simulink subsystem "PvtSubSys_VSM_SCM"  (R2020b)
settings: Solver=VariableStepAuto  StartTime=0.0  StopTime=10.0  RelTol=1e-3
undefined symbols (not defined in the file): P_Global_VehicleWidthMin_m, P_VSM_LDW_State_Param_LaneTime, P_VSM_LDW_State_Param_Speed, P_VSM_LKA_State_Param_Offset, P_VSM_LSMC_SampleTime
libraries: simulink x45
(part 1 of 3)
settings Model: Creator=GW00199575  LastModifiedBy=GW00201118

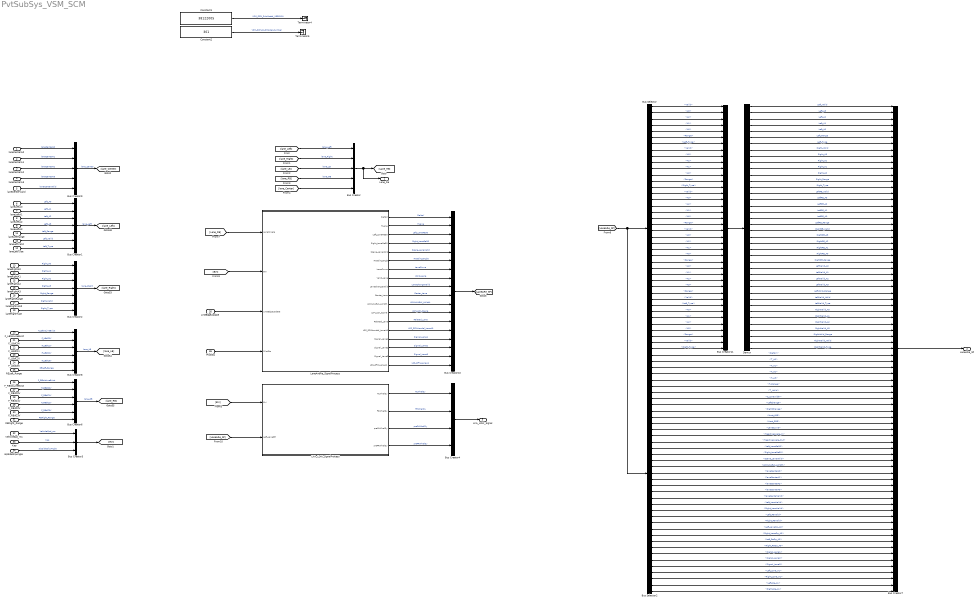
== system PvtSubSys_VSM_SCM ==
  laneCenterA0 : Inport
  laneCenterA1 : Inport  Port=2
  laneCenterA2 : Inport  Port=3
  laneCenterA3 : Inport  Port=4
  laneCenterValid : Inport  Port=5
  laneLeftA0 : Inport  Port=6
  laneLeftA1 : Inport  Port=7
  laneLeftA2 : Inport  Port=8
  laneLeftA3 : Inport  Port=9
  laneLeftValid : Inport  Port=10
  laneLeftRange : Inport  Port=11
  laneLeftType : Inport  Port=12
  laneRightA0 : Inport  Port=13
  laneRightA1 : Inport  Port=14
  laneRightA2 : Inport  Port=15
  laneRightA3 : Inport  Port=16
  laneRightValid : Inport  Port=17
  laneRightRange : Inport  Port=18
  laneRightType : Inport  Port=19
  F_LBbIsLineExist : Inport  Port=20
  F_LBdC0V : Inport  Port=21
  F_LBdC1V : Inport  Port=22
  F_LBdC2V : Inport  Port=23
  F_LBdC3V : Inport  Port=24
  RELeft_Range : Inport  Port=25
  F_RBbIsLineExist : Inport  Port=26
  F_RBdC0V : Inport  Port=27
  F_RBdC1V : Inport  Port=28
  F_RBdC2V : Inport  Port=29
  F_RBdC3V : Inport  Port=30
  RERight_Range : Inport  Port=31
  VehicleSpd_ms : Inport  Port=32
  Kap : Inport  Port=33
  alpSideSlipAngle : Inport  Port=34
  LIneEdgeUpdate : Inport  Port=35
  PilotSts : Inport  Port=36
  Bus Creator : BusCreator  Inputs=5
  Bus Creator1 : BusCreator  Inputs=7
  Bus Creator10 : BusCreator  Inputs=18
  Bus Creator11 : BusCreator  Inputs=40
  Bus Creator2 : BusCreator  Inputs=7
  Bus Creator3 : BusCreator  Inputs=3
  Bus Creator4 : BusCreator  Inputs=4
  Bus Creator6 : BusCreator  Inputs=6
  Bus Creator7 : BusCreator  Inputs=79
  Bus Creator8 : BusCreator  Inputs=6
  Bus Creator9 : BusCreator  Inputs=5
  Bus Selector : BusSelector  OutputSignals=HLane.Left_Lane.Valid,HLane.Left_Lane.A3,HLane.Left_Lane.A2,HLane.Left_Lane.A1,HLane.Left_Lane.A0,HLane.Left_Lane.Range,HLane.Left_Lane.Left_Type,HLane.Right_Lane.Valid,HLane.Right_Lane.A3,HLane.Right_Lane.A2,HLane.Right_Lane.A1,HLane.Right_Lane.A0,HLane.Right_Lane.Range,HLane.Right_Lane.Right_Type,HLane.Left_RE.Valid,HLane.Left_RE.A3,HLane.Left_RE.A2,HLane.Left_RE.A1,HLane.Left_RE.A0,HLane.Left_RE.Range,HLane.Right_RE.Valid,HLane.Right_RE.A3,HLane.Right_RE.A2,HLane.Right_RE.A1,HLane.Right_RE.A0,HLane.Right_RE.Range,Valid_Lane.Left_ValidLane.A0,Valid_Lane.Left_ValidLane.A1,Valid_Lane.Left_ValidLane.A2,Valid_Lane.Left_ValidLane.A3,Valid_Lane.Left_ValidLane.Range,Valid_Lane.Left_ValidLane.Valid,Valid_Lane.Left_ValidLane.Left_Type,Valid_Lane.Right_ValidLane.A0,Valid_Lane.Right_ValidLane.A1,Valid_Lane.Right_ValidLane.A2,Valid_Lane.Right_ValidLane.A3,Valid_Lane.Right_ValidLane.Range,Valid_Lane.Right_ValidLane.Valid,Valid_Lane.Right_ValidLane.Right_Type
  Bus Selector2 : BusSelector  OutputSignals=DeltaY,Center_Lane.T_A0,Center_Lane.T_A1,Center_Lane.T_A2,Center_Lane.T_A3,Center_Lane.T_Range,Center_Lane.T_Valid,Center_Lane.C_Lanewidth,LaneChangeValid.LeftChange,LaneChangeValid.RightChange,Valid_Lane.Host_LRE,Valid_Lane.Host_RRE,LaneCurve,Headingangle.HeadingAngle_In,Headingangle.HeadingAngle_Out,Left_LaneRe30,Right_LaneRe30,Scene_LaneValid,LDWLKAELK_LWidth,LSM_LCK_CLane.laneCenterA0,LSM_LCK_CLane.laneCenterA1,LSM_LCK_CLane.laneCenterA2,LSM_LCK_CLane.laneCenterA3,LSM_LCK_CLane.laneCenterValid,Related_Lane.Left_LaneValid,Related_Lane.Right_LaneValid,Related_Lane.Left_ReValid,Related_Lane.Right_ReValid,LSS_RFMHandel_LaneA0.Left_LaneOp_A0,LSS_RFMHandel_LaneA0.Right_LaneOp_A0,LSS_RFMHandel_LaneA0.Left_ReOp_A0,LSS_RFMHandel_LaneA0.Right_ReOp_A0,Signal_Lane1,Signal_Lane2,Signal_Lane3,LSS_RFM_LaneA1.Left_Lane_A1,LSS_RFM_LaneA1.Right_Lane_A1,LSS_RFM_LaneA1.Left_Re_A1,LSS_RFM_LaneA1.Right_Re_A1
  Constant1 : Constant  Value=38122005  OutDataTypeStr=uint32
  Constant2 : Constant  Value=301  OutDataTypeStr=uint16
  Demux : Demux  Outputs=40  BusSelectionMode=on
  LKA_LDW_SignalProcess : Subsystem
  LaneAndRe_SignalProcess : Subsystem
  Terminator4 : Terminator
  Terminator5 : Terminator
  Lane_Re : Outport
  LaneARe_SP : Outport  Port=2
  LKA_LDW_Signal : Outport  Port=3
  wires:
  Bus Selector2/39 -> Bus Creator7/79  "<Right_Re_A1>"
  Bus Selector2/38 -> Bus Creator7/78  "<Left_Re_A1>"
  Bus Selector2/37 -> Bus Creator7/77  "<Right_Lane_A1>"
  Bus Selector2/36 -> Bus Creator7/76  "<Left_Lane_A1>"
  Bus Selector2/35 -> Bus Creator7/75  "<Signal_Lane3>"
  Bus Selector2/34 -> Bus Creator7/74  "<Signal_Lane2>"
  Bus Selector2/33 -> Bus Creator7/73  "<Signal_Lane1>"
  Bus Selector2/32 -> Bus Creator7/72  "<Right_ReOp_A0>"
  Bus Selector2/31 -> Bus Creator7/71  "<Left_ReOp_A0>"
  Bus Selector2/30 -> Bus Creator7/70  "<Right_LaneOp_A0>"
  Bus Selector2/29 -> Bus Creator7/69  "<Left_LaneOp_A0>"
  Bus Selector2/28 -> Bus Creator7/68  "<Right_ReValid>"
  Bus Selector2/27 -> Bus Creator7/67  "<Left_ReValid>"
  Bus Selector2/26 -> Bus Creator7/66  "<Right_LaneValid>"
  Bus Selector2/25 -> Bus Creator7/65  "<Left_LaneValid>"
  Bus Selector2/24 -> Bus Creator7/64  "<laneCenterValid>"
  LaneAndRe_SignalProcess/18(LSS_RFM_LaneA1) -> Bus Creator10/18  "LSS_RFM_LaneA1"
  LaneAndRe_SignalProcess/17(Signal_Lane3) -> Bus Creator10/17  "Signal_Lane3"
  LaneAndRe_SignalProcess/16(Signal_Lane2) -> Bus Creator10/16  "Signal_Lane2"
  LaneAndRe_SignalProcess/15(Signal_Lane1) -> Bus Creator10/15  "Signal_Lane1"
  LaneAndRe_SignalProcess/14(LSS_RFMHandel_LaneA0) -> Bus Creator10/14  "LSS_RFMHandel_LaneA0"
  LaneAndRe_SignalProcess/13(Related_Lane) -> Bus Creator10/13  "Related_Lane"
  LaneAndRe_SignalProcess/12(LSM_LCK_CLane) -> Bus Creator10/12  "LSM_LCK_CLane"
  LaneAndRe_SignalProcess/11(LDWLKAELK_LWidth) -> Bus Creator10/11  "LDWLKAELK_LWidth"
  PilotSts/1 -> LaneAndRe_SignalProcess/4(PilotSts)
  [LaneARe_SP] -> LKA_LDW_SignalProcess/2(Left_LaneRE)
  [lane_Center] -> Bus Creator/5
  LKA_LDW_SignalProcess/4(preFRWhelDy) -> Bus Creator4/4  "preFRWhelDy"
  LKA_LDW_SignalProcess/3(preFLWhelDy) -> Bus Creator4/3  "preFLWhelDy"
  LKA_LDW_SignalProcess/2(FRWhelDy) -> Bus Creator4/2  "FRWhelDy"
  LKA_LDW_SignalProcess/1(FLWhelDy) -> Bus Creator4/1  "FLWhelDy"
  [EVI] -> LKA_LDW_SignalProcess/1(Evi)
  laneCenterValid/1 -> Bus Creator9/5  "laneCenterValid"
  Bus Creator9/1 -> [lane_Center]  "lane_Center"
  laneCenterA3/1 -> Bus Creator9/4  "laneCenterA3"
  laneCenterA0/1 -> Bus Creator9/1  "laneCenterA0"
  laneCenterA1/1 -> Bus Creator9/2  "laneCenterA1"
  laneCenterA2/1 -> Bus Creator9/3  "laneCenterA2"
  [EVI] -> LaneAndRe_SignalProcess/2(EVI)
  LIneEdgeUpdate/1 -> LaneAndRe_SignalProcess/3(LIneEdgeUpdate)
  [Lane_RE] -> LaneAndRe_SignalProcess/1(LaneSingle)
  LaneAndRe_SignalProcess/7(LaneCurve) -> Bus Creator10/7  "LaneCurve"
  LaneAndRe_SignalProcess/6(Headingangle) -> Bus Creator10/6  "Headingangle"
  LaneAndRe_SignalProcess/5(Scene_LaneValid) -> Bus Creator10/5  "Scene_LaneValid"
  Bus Creator10/1 -> [LaneARe_SP]
  LaneAndRe_SignalProcess/10(Center_Lane) -> Bus Creator10/10  "Center_Lane"
  LaneAndRe_SignalProcess/1(DeltaY) -> Bus Creator10/1  "DeltaY"
  LaneAndRe_SignalProcess/3(Left_LaneRe30) -> Bus Creator10/3  "Left_LaneRe30"
  LaneAndRe_SignalProcess/2(HLane) -> Bus Creator10/2  "HLane"
  LaneAndRe_SignalProcess/8(Valid_Lane) -> Bus Creator10/8  "Valid_Lane"
  LaneAndRe_SignalProcess/4(Right_LaneRe30) -> Bus Creator10/4  "Right_LaneRe30"
  LaneAndRe_SignalProcess/9(LaneChangeValid) -> Bus Creator10/9  "LaneChangeValid"
  laneRightType/1 -> Bus Creator2/7  "Right_Type"
  laneLeftType/1 -> Bus Creator1/7  "Left_Type"
  Bus Creator4/1 -> LKA_LDW_Signal/1
  Bus Creator3/1 -> [EVI]
  alpSideSlipAngle/1 -> Bus Creator3/3  "alpSideSlipAngle"
  Kap/1 -> Bus Creator3/2  "Kap"
  VehicleSpd_ms/1 -> Bus Creator3/1  "VehicleSpd_ms"
  Bus Creator/1 -> Lane_Re/1, [Lane_RE]
  [lane_RB] -> Bus Creator/4  "lane_RB"
  [lane_LB] -> Bus Creator/3  "lane_LB"
  [lane_Right] -> Bus Creator/2  "lane_Right"
  [lane_Left] -> Bus Creator/1  "lane_Left"
  Bus Creator6/1 -> [lane_RB]  "lane_RB"
  Bus Creator8/1 -> [lane_LB]  "lane_LB"
  Bus Creator2/1 -> [lane_Right]  "lane_Right"
  Bus Creator1/1 -> [lane_Left]  "lane_Left"
  RERight_Range/1 -> Bus Creator6/6  "RERight_Range"
  F_RBdC3V/1 -> Bus Creator6/5  "F_RBdC3V"
  F_RBdC2V/1 -> Bus Creator6/4  "F_RBdC2V"
  F_RBdC1V/1 -> Bus Creator6/3  "F_RBdC1V"
  F_RBdC0V/1 -> Bus Creator6/2  "F_RBdC0V"
  F_RBbIsLineExist/1 -> Bus Creator6/1  "F_RBbIsLineExist"
  RELeft_Range/1 -> Bus Creator8/6  "RELeft_Range"
  F_LBdC3V/1 -> Bus Creator8/5  "F_LBdC3V"
  F_LBdC2V/1 -> Bus Creator8/4  "F_LBdC2V"
  F_LBdC1V/1 -> Bus Creator8/3  "F_LBdC1V"
  F_LBdC0V/1 -> Bus Creator8/2  "F_LBdC0V"
  F_LBbIsLineExist/1 -> Bus Creator8/1  "F_LBbIsLineExist"
  laneRightValid/1 -> Bus Creator2/6  "Right_Valid"
  laneRightRange/1 -> Bus Creator2/5  "Right_Range"
  laneRightA0/1 -> Bus Creator2/1  "Right_A0"
  laneRightA3/1 -> Bus Creator2/4  "Right_A3"
  laneRightA1/1 -> Bus Creator2/2  "Right_A1"
  laneRightA2/1 -> Bus Creator2/3  "Right_A2"
  laneLeftValid/1 -> Bus Creator1/6  "Left_Valid"
  laneLeftRange/1 -> Bus Creator1/5  "Left_Range"
  laneLeftA2/1 -> Bus Creator1/3  "Left_A2"
  laneLeftA3/1 -> Bus Creator1/4  "Left_A3"
  laneLeftA1/1 -> Bus Creator1/2  "Left_A1"
  laneLeftA0/1 -> Bus Creator1/1  "Left_A0"
  [LaneARe_SP] -> Bus Selector/1, Bus Selector2/1
  Bus Creator7/1 -> LaneARe_SP/1
  Bus Selector/1 -> Bus Creator11/1  "<Valid>"
  Bus Selector/2 -> Bus Creator11/2  "<A3>"
  Bus Selector/3 -> Bus Creator11/3  "<A2>"
  Bus Selector/4 -> Bus Creator11/4  "<A1>"
  Bus Selector/5 -> Bus Creator11/5  "<A0>"
  Bus Selector/6 -> Bus Creator11/6  "<Range>"
  Bus Selector/7 -> Bus Creator11/7  "<Left_Type>"
  Bus Selector/8 -> Bus Creator11/8  "<Valid>"
  Bus Selector/9 -> Bus Creator11/9  "<A3>"
  Bus Selector/10 -> Bus Creator11/10  "<A2>"
  Bus Selector/11 -> Bus Creator11/11  "<A1>"
  Bus Selector/12 -> Bus Creator11/12  "<A0>"
  Bus Selector/13 -> Bus Creator11/13  "<Range>"
  Bus Selector/14 -> Bus Creator11/14  "<Right_Type>"
  Bus Selector/15 -> Bus Creator11/15  "<Valid>"
  Bus Selector/16 -> Bus Creator11/16  "<A3>"
  Bus Selector/17 -> Bus Creator11/17  "<A2>"
  Bus Selector/18 -> Bus Creator11/18  "<A1>"
  Bus Selector/19 -> Bus Creator11/19  "<A0>"
  Bus Selector/20 -> Bus Creator11/20  "<Range>"
  Bus Selector/21 -> Bus Creator11/21  "<Valid>"
  Bus Selector/22 -> Bus Creator11/22  "<A3>"
  Bus Selector/23 -> Bus Creator11/23  "<A2>"
  Bus Selector/24 -> Bus Creator11/24  "<A1>"
  Bus Selector/25 -> Bus Creator11/25  "<A0>"
  Bus Selector/26 -> Bus Creator11/26  "<Range>"
  Bus Selector/27 -> Bus Creator11/27  "<A0>"
  Bus Selector/28 -> Bus Creator11/28  "<A1>"
  Bus Selector/29 -> Bus Creator11/29  "<A2>"
  Bus Selector/30 -> Bus Creator11/30  "<A3>"
  Bus Selector/31 -> Bus Creator11/31  "<Range>"
  Bus Selector/32 -> Bus Creator11/32  "<Valid>"
  Bus Selector/33 -> Bus Creator11/33  "<Left_Type>"
  Bus Selector/34 -> Bus Creator11/34  "<A0>"
  Bus Selector/35 -> Bus Creator11/35  "<A1>"
  Bus Selector/36 -> Bus Creator11/36  "<A2>"
  Bus Selector/37 -> Bus Creator11/37  "<A3>"
  Bus Selector/38 -> Bus Creator11/38  "<Range>"
  Bus Selector/39 -> Bus Creator11/39  "<Valid>"
  Bus Selector/40 -> Bus Creator11/40  "<Right_Type>"
  Bus Creator11/1 -> Demux/1
  Demux/1 -> Bus Creator7/1  "Left_Valid"
  Demux/2 -> Bus Creator7/2  "Left_A3"
  Demux/3 -> Bus Creator7/3  "Left_A2"
  Demux/4 -> Bus Creator7/4  "Left_A1"
  Demux/5 -> Bus Creator7/5  "Left_A0"
  Demux/6 -> Bus Creator7/6  "Left_Range"
  Demux/7 -> Bus Creator7/7  "Left_Type"
  Demux/8 -> Bus Creator7/8  "Right_Valid"
  Demux/9 -> Bus Creator7/9  "Right_A3"
  Demux/10 -> Bus Creator7/10  "Right_A2"
  Demux/11 -> Bus Creator7/11  "Right_A1"
  Demux/12 -> Bus Creator7/12  "Right_A0"
  Demux/13 -> Bus Creator7/13  "Right_Range"
  Demux/14 -> Bus Creator7/14  "Right_Type"
  Demux/15 -> Bus Creator7/15  "LeftRE_Valid"
  Demux/16 -> Bus Creator7/16  "LeftRE_A3"
  Demux/17 -> Bus Creator7/17  "LeftRE_A2"
  Demux/18 -> Bus Creator7/18  "LeftRE_A1"
  Demux/19 -> Bus Creator7/19  "LeftRE_A0"
  Demux/20 -> Bus Creator7/20  "LeftRE_Range"
  Demux/21 -> Bus Creator7/21  "RightRE_Valid"
  Demux/22 -> Bus Creator7/22  "RightRE_A3"
  Demux/23 -> Bus Creator7/23  "RightRE_A2"
  Demux/24 -> Bus Creator7/24  "RightRE_A1"
  Demux/25 -> Bus Creator7/25  "RightRE_A0"
  Demux/26 -> Bus Creator7/26  "RightRE_Range"
  Demux/27 -> Bus Creator7/27  "LeftValid_A0"
  Demux/28 -> Bus Creator7/28  "LeftValid_A1"
  Demux/29 -> Bus Creator7/29  "LeftValid_A2"
  Demux/30 -> Bus Creator7/30  "LeftValid_A3"
  Demux/31 -> Bus Creator7/31  "LeftValid_Range"
  Demux/32 -> Bus Creator7/32  "LeftValid_Valid"
  Demux/33 -> Bus Creator7/33  "LeftValid_Type"
  Demux/34 -> Bus Creator7/34  "RightValid_A0"
  Demux/35 -> Bus Creator7/35  "RightValid_A1"
  Demux/36 -> Bus Creator7/36  "RightValid_A2"
  Demux/37 -> Bus Creator7/37  "RightValid_A3"
  Demux/38 -> Bus Creator7/38  "RightValid_Range"
  Demux/39 -> Bus Creator7/39  "RightValid_Valid"
  Demux/40 -> Bus Creator7/40  "RightValid_Type"
  Bus Selector2/1 -> Bus Creator7/41  "<DeltaY>"
  Bus Selector2/2 -> Bus Creator7/42  "<T_A0>"
  Bus Selector2/3 -> Bus Creator7/43  "<T_A1>"
  Bus Selector2/4 -> Bus Creator7/44  "<T_A2>"
  Bus Selector2/5 -> Bus Creator7/45  "<T_A3>"
  Bus Selector2/6 -> Bus Creator7/46  "<T_Range>"
  Bus Selector2/7 -> Bus Creator7/47  "<T_Valid>"
  Bus Selector2/8 -> Bus Creator7/48  "<C_Lanewidth>"
  Bus Selector2/9 -> Bus Creator7/49  "<LeftChange>"
  Bus Selector2/10 -> Bus Creator7/50  "<RightChange>"
  Bus Selector2/11 -> Bus Creator7/51  "<Host_LRE>"
  Bus Selector2/12 -> Bus Creator7/52  "<Host_RRE>"
  Bus Selector2/13 -> Bus Creator7/53  "<LaneCurve>"
  Bus Selector2/14 -> Bus Creator7/54  "<HeadingAngle_In>"
  Bus Selector2/15 -> Bus Creator7/55  "<HeadingAngle_Out>"
  Bus Selector2/16 -> Bus Creator7/56  "<Left_LaneRe30>"
  Bus Selector2/17 -> Bus Creator7/57  "<Right_LaneRe30>"
  Bus Selector2/18 -> Bus Creator7/58  "<Scene_LaneValid>"
  Bus Selector2/19 -> Bus Creator7/59  "<LDWLKAELK_LWidth>"
  Bus Selector2/20 -> Bus Creator7/60  "<laneCenterA0>"
  Bus Selector2/21 -> Bus Creator7/61  "<laneCenterA1>"
  Bus Selector2/22 -> Bus Creator7/62  "<laneCenterA2>"
  Bus Selector2/23 -> Bus Creator7/63  "<laneCenterA3>"
  Constant1/1 -> Terminator4/1  "VSM_SCM_SubModel_VERSION"
  Constant2/1 -> Terminator5/1  "VSM_SCM_SubModel_Number"

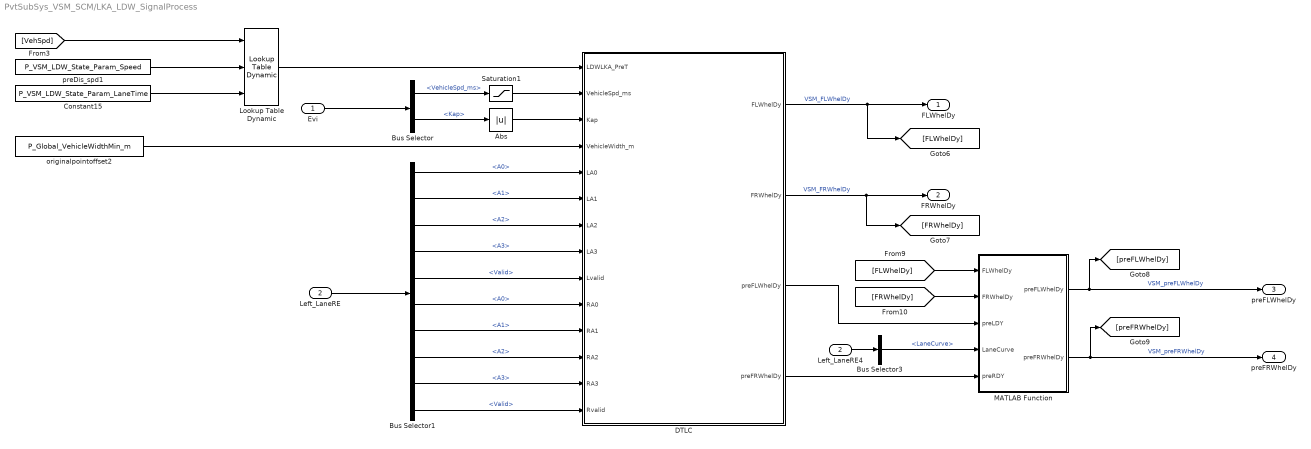
== system PvtSubSys_VSM_SCM/LKA_LDW_SignalProcess ==
  Evi : Inport
  Left_LaneRE : Inport  Port=2
  Abs : Abs
  Bus Selector : BusSelector  OutputSignals=VehicleSpd_ms,Kap
  Bus Selector1 : BusSelector  OutputSignals=Valid_Lane.Left_ValidLane.A0,Valid_Lane.Left_ValidLane.A1,Valid_Lane.Left_ValidLane.A2,Valid_Lane.Left_ValidLane.A3,Valid_Lane.Left_ValidLane.Valid,Valid_Lane.Right_ValidLane.A0,Valid_Lane.Right_ValidLane.A1,Valid_Lane.Right_ValidLane.A2,Valid_Lane.Right_ValidLane.A3,Valid_Lane.Right_ValidLane.Valid
  Bus Selector3 : BusSelector  OutputSignals=LaneCurve
  Constant15 : Constant  Value=P_VSM_LDW_State_Param_LaneTime
  DTLC : MATLAB Function  Description=%Lane inside is positive,outside is negitive  TreatAsAtomicUnit=on
  Left_LaneRE4 : InportShadow  Port=2
  Lookup Table Dynamic : simulink/Lookup Tables/Lookup Table Dynamic  LookUpMeth=Interpolation-Use End Values  OutDataType=fixdt('double')  OutScaling=[]  OutputDataTypeScalingMode=Specify via dialog  OutDataTypeStr=double  DoSatur=off
  MATLAB Function : MATLAB Function  TreatAsAtomicUnit=on
  Saturation1 : Saturate  UpperLimit=200  LowerLimit=0.001
  originalpointoffset2 : Constant  Value=P_Global_VehicleWidthMin_m
  preDis_spd1 : Constant  Value=P_VSM_LDW_State_Param_Speed
  FLWhelDy : Outport
  FRWhelDy : Outport  Port=2
  preFLWhelDy : Outport  Port=3
  preFRWhelDy : Outport  Port=4
  wires:
  Abs/1 -> DTLC/3(Kap)
  Bus Selector1/10 -> DTLC/14(Rvalid)  "<Valid>"
  Bus Selector1/9 -> DTLC/13(RA3)  "<A3>"
  Bus Selector1/8 -> DTLC/12(RA2)  "<A2>"
  Bus Selector1/7 -> DTLC/11(RA1)  "<A1>"
  Bus Selector1/6 -> DTLC/10(RA0)  "<A0>"
  originalpointoffset2/1 -> DTLC/4(VehicleWidth_m)
  Bus Selector1/5 -> DTLC/9(Lvalid)  "<Valid>"
  Bus Selector1/4 -> DTLC/8(LA3)  "<A3>"
  Bus Selector1/3 -> DTLC/7(LA2)  "<A2>"
  Bus Selector1/2 -> DTLC/6(LA1)  "<A1>"
  Bus Selector1/1 -> DTLC/5(LA0)  "<A0>"
  Left_LaneRE/1 -> Bus Selector1/1
  Bus Selector/2 -> Abs/1  "<Kap>"
  Bus Selector/1 -> Saturation1/1  "<VehicleSpd_ms>"
  Evi/1 -> Bus Selector/1
  DTLC/2(FRWhelDy) -> [FRWhelDy], FRWhelDy/1  "VSM_FRWhelDy"
  DTLC/1(FLWhelDy) -> [FLWhelDy], FLWhelDy/1  "VSM_FLWhelDy"
  Constant15/1 -> Lookup Table Dynamic/3
  [VehSpd] -> Lookup Table Dynamic/1
  preDis_spd1/1 -> Lookup Table Dynamic/2
  Saturation1/1 -> DTLC/2(VehicleSpd_ms)
  Lookup Table Dynamic/1 -> DTLC/1(LDWLKA_PreT)
  DTLC/3(preFLWhelDy) -> MATLAB Function/3(preLDY)
  DTLC/4(preFRWhelDy) -> MATLAB Function/5(preRDY)
  MATLAB Function/2(preFRWhelDy) -> [preFRWhelDy], preFRWhelDy/1  "VSM_preFRWhelDy"
  MATLAB Function/1(preFLWhelDy) -> [preFLWhelDy], preFLWhelDy/1  "VSM_preFLWhelDy"
  [FLWhelDy] -> MATLAB Function/1(FLWhelDy)
  [FRWhelDy] -> MATLAB Function/2(FRWhelDy)
  Left_LaneRE4/1 -> Bus Selector3/1
  Bus Selector3/1 -> MATLAB Function/4(LaneCurve)  "<LaneCurve>"

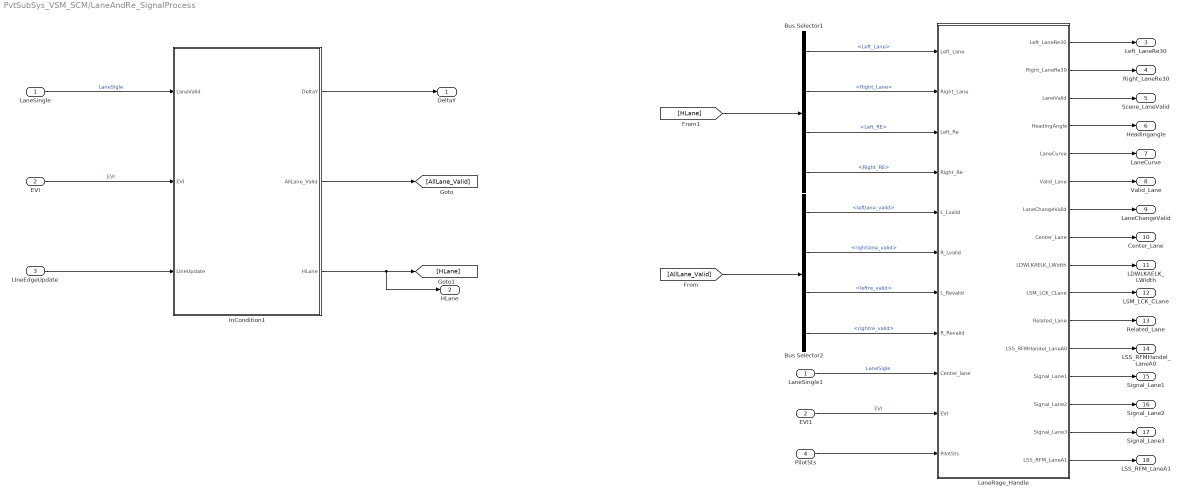
== system PvtSubSys_VSM_SCM/LaneAndRe_SignalProcess ==
  LaneSingle : Inport
  EVI : Inport  Port=2
  LIneEdgeUpdate : Inport  Port=3
  PilotSts : Inport  Port=4
  Bus Selector1 : BusSelector  OutputSignals=Left_Lane,Right_Lane,Left_RE,Right_RE
  Bus Selector2 : BusSelector  OutputSignals=leftlane_valid,rightlane_valid,leftre_valid,rightre_valid
  EVI1 : InportShadow  Port=2
  InCondition1 : Subsystem
  LaneRage_Handle : Subsystem
  LaneSingle1 : InportShadow
  DeltaY : Outport
  HLane : Outport  Port=2
  Left_LaneRe30 : Outport  Port=3
  Right_LaneRe30 : Outport  Port=4
  Scene_LaneValid : Outport  Port=5
  Headingangle : Outport  Port=6
  LaneCurve : Outport  Port=7
  Valid_Lane : Outport  Port=8
  LaneChangeValid : Outport  Port=9
  Center_Lane : Outport  Port=10
  LDWLKAELK_LWidth : Outport  Port=11
  LSM_LCK_CLane : Outport  Port=12
  Related_Lane : Outport  Port=13
  LSS_RFMHandel_LaneA0 : Outport  Port=14
  Signal_Lane1 : Outport  Port=15
  Signal_Lane2 : Outport  Port=16
  Signal_Lane3 : Outport  Port=17
  LSS_RFM_LaneA1 : Outport  Port=18
  wires:
  EVI/1 -> InCondition1/2(EVI)  "EVI"
  LaneSingle/1 -> InCondition1/1(LaneValid)  "LaneSigle"
  Bus Selector1/2 -> LaneRage_Handle/2(Right_Lane)  "<Right_Lane>"
  Bus Selector2/2 -> LaneRage_Handle/6(R_Lvalid)  "<rightlane_valid>"
  Bus Selector1/3 -> LaneRage_Handle/3(Left_Re)  "<Left_RE>"
  Bus Selector2/1 -> LaneRage_Handle/5(L_Lvalid)  "<leftlane_valid>"
  LIneEdgeUpdate/1 -> InCondition1/3(LineUpdate)
  Bus Selector1/1 -> LaneRage_Handle/1(Left_Lane)  "<Left_Lane>"
  LaneRage_Handle/3(LaneValid) -> Scene_LaneValid/1
  Bus Selector2/3 -> LaneRage_Handle/7(L_Revalid)  "<leftre_valid>"
  Bus Selector2/4 -> LaneRage_Handle/8(R_Revalid)  "<rightre_valid>"
  Bus Selector1/4 -> LaneRage_Handle/4(Right_Re)  "<Right_RE>"
  InCondition1/2(AllLane_Valid) -> [AllLane_Valid]
  InCondition1/3(HLane) -> HLane/1, [HLane]
  InCondition1/1(DeltaY) -> DeltaY/1
  [AllLane_Valid] -> Bus Selector2/1
  [HLane] -> Bus Selector1/1
  LaneRage_Handle/4(HeadingAngle) -> Headingangle/1
  LaneRage_Handle/5(LaneCurve) -> LaneCurve/1
  LaneRage_Handle/6(Valid_Lane) -> Valid_Lane/1
  LaneRage_Handle/7(LaneChangeValid) -> LaneChangeValid/1
  LaneRage_Handle/1(Left_LaneRe30) -> Left_LaneRe30/1
  LaneRage_Handle/2(Right_LaneRe30) -> Right_LaneRe30/1
  LaneRage_Handle/8(Center_Lane) -> Center_Lane/1
  LaneSingle1/1 -> LaneRage_Handle/9(Center_lane)  "LaneSigle"
  EVI1/1 -> LaneRage_Handle/10(EVI)  "EVI"
  PilotSts/1 -> LaneRage_Handle/11(PilotSts)
  LaneRage_Handle/9(LDWLKAELK_LWidth) -> LDWLKAELK_LWidth/1
  LaneRage_Handle/10(LSM_LCK_CLane) -> LSM_LCK_CLane/1
  LaneRage_Handle/11(Related_Lane) -> Related_Lane/1
  LaneRage_Handle/12(LSS_RFMHandel_LaneA0) -> LSS_RFMHandel_LaneA0/1
  LaneRage_Handle/13(Signal_Lane1) -> Signal_Lane1/1
  LaneRage_Handle/14(Signal_Lane2) -> Signal_Lane2/1
  LaneRage_Handle/15(Signal_Lane3) -> Signal_Lane3/1
  LaneRage_Handle/16(LSS_RFM_LaneA1) -> LSS_RFM_LaneA1/1

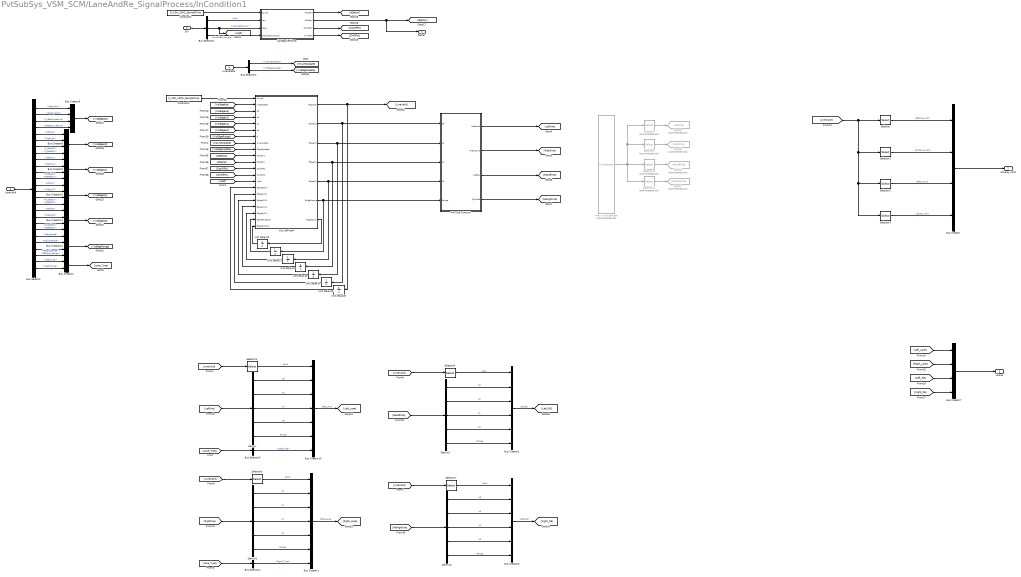
== system PvtSubSys_VSM_SCM/LaneAndRe_SignalProcess/InCondition1 ==
  LaneValid : Inport
  EVI : Inport  Port=2
  LineUpdate : Inport  Port=3
  Bus Creator{,5..7,9..12} (8 alike) : BusCreator  Inputs=4
  Bus Creator1 : BusCreator  Inputs=7
  Bus Creator13 : BusCreator  Inputs=7
  Bus Creator2 : BusCreator  Inputs=6
  Bus Creator3 : BusCreator  Inputs=6
  Bus Creator4 : BusCreator  Inputs=2
  Bus Selector : BusSelector  OutputSignals=lane_Left.Left_Valid,lane_Right.Right_Valid,lane_LB.F_LBbIsLineExist,lane_RB.F_RBbIsLineExist,lane_Left.Left_A0,lane_Right.Right_A0,lane_LB.F_LBdC0V,lane_RB.F_RBdC0V,lane_Left.Left_A1,lane_Right.Right_A1,lane_LB.F_LBdC1V,lane_RB.F_RBdC1V,lane_Left.Left_A2,lane_Right.Right_A2,lane_LB.F_LBdC2V,lane_RB.F_RBdC2V,lane_Left.Left_A3,lane_Right.Right_A3,lane_LB.F_LBdC3V,lane_RB.F_RBdC3V,lane_Left.Left_Range,lane_Right.Right_Range,lane_LB.RELeft_Range,lane_RB.RERight_Range,lane_Left.Left_Type,lane_Right.Right_Type
  Bus Selector1 : BusSelector  OutputSignals=Kap,VehicleSpd_ms,alpSideSlipAngle
  Bus Selector2 : BusSelector  OutputSignals=VisLaneUpdate,VisEdgeUpdate
  Bus Selector3 : BusSelector  OutputSignals=Left_Type
  Bus Selector4 : BusSelector  OutputSignals=Right_Type
  CalcEgoVehMove : MATLAB Function  TreatAsAtomicUnit=on
  Constant2 : Constant  Value=P_VSM_LSMC_SampleTime
  Constant4 : Constant  Value=P_VSM_LSMC_SampleTime
  Demux{,1..3} (4 alike) : Demux  Outputs=5
  Goto30 : Goto  Commented=on  GotoTag=Leftline
  Goto35 : Goto  Commented=on  GotoTag=Rightline
  Goto36 : Goto  Commented=on  GotoTag=ReLeftline
  Goto37 : Goto  Commented=on  GotoTag=ReRightline
  MATLAB Function : MATLAB Function  TreatAsAtomicUnit=on
  Matrix Concatenate : Concatenate  Commented=on  NumInputs=5  Mode=Multidimensional array  ConcatenateDimension=2
  Selector : Selector  InputPortWidth=4  IndexOptions=Index vector (dialog)  Indices=1  OutputSizes=1
  Selector1 : Selector  InputPortWidth=4  IndexOptions=Index vector (dialog)  Indices=2  OutputSizes=1
  Selector10 : Selector  Commented=on  NumberOfDimensions=2  InputPortWidth=4  IndexOptions=Index vector (dialog),Select all  Indices=3,1  OutputSizes=1,1
  Selector11 : Selector  Commented=on  NumberOfDimensions=2  InputPortWidth=4  IndexOptions=Index vector (dialog),Select all  Indices=4,1  OutputSizes=1,1
  Selector2 : Selector  InputPortWidth=4  IndexOptions=Index vector (dialog)  Indices=3  OutputSizes=1
  Selector3 : Selector  InputPortWidth=4  IndexOptions=Index vector (dialog)  Indices=4  OutputSizes=1
  Selector4 : Selector  InputPortWidth=4  IndexOptions=Index vector (dialog)  Indices=1  OutputSizes=1
  Selector5 : Selector  InputPortWidth=4  IndexOptions=Index vector (dialog)  Indices=2  OutputSizes=1
  Selector6 : Selector  InputPortWidth=4  IndexOptions=Index vector (dialog)  Indices=3  OutputSizes=1
  Selector7 : Selector  InputPortWidth=4  IndexOptions=Index vector (dialog)  Indices=4  OutputSizes=1
  Selector8 : Selector  Commented=on  NumberOfDimensions=2  InputPortWidth=4  IndexOptions=Index vector (dialog),Select all  Indices=1,1  OutputSizes=1,1
  Selector9 : Selector  Commented=on  NumberOfDimensions=2  InputPortWidth=4  IndexOptions=Index vector (dialog),Select all  Indices=2,1  OutputSizes=1,1
  Unit Delay20 : UnitDelay  InitialCondition=[5;5;5;5]  SampleTime=-1  HasFrameUpgradeWarning=on
  Unit Delay{21..26} (6 alike) : UnitDelay  InitialCondition=zeros(4,1)  SampleTime=-1  HasFrameUpgradeWarning=on
  VisLineFilter4 : MATLAB Function  TreatAsAtomicUnit=on
  DeltaY : Outport
  AllLane_Valid : Outport  Port=2
  HLane : Outport  Port=3
  wires:
  Constant4/1 -> VisLineFilter4/1(tCycle)
  Constant2/1 -> CalcEgoVehMove/1(tCycle)
  Bus Selector4/1 -> Bus Creator1/7  "<Right_Type>"
  [Lane_Type] -> Bus Selector4/1
  Bus Selector3/1 -> Bus Creator13/7  "<Left_Type>"
  [Lane_Type] -> Bus Selector3/1
  Bus Creator4/1 -> [Lane_Type]
  Bus Selector/25 -> Bus Creator4/1  "<Left_Type>"
  Bus Selector/26 -> Bus Creator4/2  "<Right_Type>"
  Demux3/5 -> Bus Creator3/6  "Range"
  Demux3/4 -> Bus Creator3/5  "A0"
  Demux3/3 -> Bus Creator3/4  "A1"
  Demux3/2 -> Bus Creator3/3  "A2"
  Demux3/1 -> Bus Creator3/2  "A3"
  Demux2/5 -> Bus Creator2/6  "Range"
  Demux2/4 -> Bus Creator2/5  "A0"
  Demux2/3 -> Bus Creator2/4  "A1"
  Demux2/2 -> Bus Creator2/3  "A2"
  Demux2/1 -> Bus Creator2/2  "A3"
  Demux1/5 -> Bus Creator1/6  "Range"
  Demux1/4 -> Bus Creator1/5  "A0"
  Demux1/3 -> Bus Creator1/4  "A1"
  Demux1/2 -> Bus Creator1/3  "A2"
  Demux1/1 -> Bus Creator1/2  "A3"
  Demux/5 -> Bus Creator13/6  "Range"
  Demux/4 -> Bus Creator13/5  "A0"
  Demux/3 -> Bus Creator13/4  "A1"
  Demux/2 -> Bus Creator13/3  "A2"
  Demux/1 -> Bus Creator13/2  "A3"
  CalcEgoVehMove/2(dDeltaY) -> [dDeltaY], DeltaY/1
  [VisEdgeUpdate] -> VisLineFilter4/9(EdgeUpdate)
  [VisLineUpdate] -> VisLineFilter4/8(LineUpdate)
  Bus Selector2/2 -> [VisEdgeUpdate]  "<VisEdgeUpdate>"
  Bus Selector2/1 -> [VisLineUpdate]  "<VisLaneUpdate>"
  LineUpdate/1 -> Bus Selector2/1
  EVI/1 -> Bus Selector1/1
  [ReRightline] -> Demux3/1
  [ReLeftline] -> Demux2/1
  [Rightline] -> Demux1/1
  [Leftline] -> Demux/1
  Selector11/1 -> Goto37/1
  Selector10/1 -> Goto36/1
  Selector9/1 -> Goto35/1
  Selector8/1 -> Goto30/1
  Matrix Concatenate/1 -> Selector10/1, Selector11/1, Selector9/1, Selector8/1
  Bus Creator/1 -> AllLane_Valid/1
  Bus Creator3/1 -> [Right_RE]  "Right_RE"
  Bus Creator2/1 -> [Left_RE]  "Left_RE"
  Bus Creator1/1 -> [Right_Lane]  "Right_Lane"
  Selector3/1 -> Bus Creator/4  "rightre_valid"
  Selector2/1 -> Bus Creator/3  "leftre_valid"
  Selector1/1 -> Bus Creator/2  "rightlane_valid"
  [LineValid] -> Selector/1, Selector2/1, Selector3/1, Selector1/1
  Selector/1 -> Bus Creator/1  "leftlane_valid"
  Bus Creator12/1 -> [VisEdgeRange]
  Bus Selector/24 -> Bus Creator12/4  "<RERight_Range>"
  Bus Selector/23 -> Bus Creator12/3  "<RELeft_Range>"
  Bus Selector/22 -> Bus Creator12/2  "<Right_Range>"
  Bus Selector/21 -> Bus Creator12/1  "<Left_Range>"
  Bus Creator9/1 -> [VisEdgeA1]
  Bus Creator6/1 -> [VisEdgeA0]
  Bus Creator10/1 -> [VisEdgeA2]
  Bus Creator11/1 -> [VisEdgeA3]
  Bus Creator5/1 -> [VisEdgeSts]
  Bus Selector/20 -> Bus Creator11/4  "<F_RBdC3V>"
  Bus Selector/19 -> Bus Creator11/3  "<F_LBdC3V>"
  Bus Selector/18 -> Bus Creator11/2  "<Right_A3>"
  Bus Selector/17 -> Bus Creator11/1  "<Left_A3>"
  Bus Selector/16 -> Bus Creator10/4  "<F_RBdC2V>"
  Bus Selector/15 -> Bus Creator10/3  "<F_LBdC2V>"
  Bus Selector/14 -> Bus Creator10/2  "<Right_A2>"
  Bus Selector/13 -> Bus Creator10/1  "<Left_A2>"
  Bus Selector/12 -> Bus Creator9/4  "<F_RBdC1V>"
  Bus Selector/11 -> Bus Creator9/3  "<F_LBdC1V>"
  Bus Selector/10 -> Bus Creator9/2  "<Right_A1>"
  Bus Selector/9 -> Bus Creator9/1  "<Left_A1>"
  Bus Selector/8 -> Bus Creator6/4  "<F_RBdC0V>"
  Bus Selector/7 -> Bus Creator6/3  "<F_LBdC0V>"
  Bus Selector/6 -> Bus Creator6/2  "<Right_A0>"
  Bus Selector/5 -> Bus Creator6/1  "<Left_A0>"
  Bus Selector/4 -> Bus Creator5/4  "<F_RBbIsLineExist>"
  Bus Selector/3 -> Bus Creator5/3  "<F_LBbIsLineExist>"
  Bus Selector/2 -> Bus Creator5/2  "<Right_Valid>"
  Bus Selector/1 -> Bus Creator5/1  "<Left_Valid>"
  [VisEdgeSts] -> VisLineFilter4/2(VisEdgeSts)
  [VisEdgeA0] -> VisLineFilter4/6(a0)
  [VisEdgeRange] -> VisLineFilter4/7(R)
  VisLineFilter4/6(EdgeRange) -> MATLAB Function/5(Range), Unit Delay21/1
  Unit Delay25/1 -> VisLineFilter4/16(EdgeA3K1)
  [SinOfPsi] -> VisLineFilter4/13(SinOfPsi)
  [VisEdgeA2] -> VisLineFilter4/4(a2)
  Unit Delay22/1 -> VisLineFilter4/19(EdgeA0K1)
  Unit Delay26/1 -> VisLineFilter4/15(EdgeStsK1)
  VisLineFilter4/7(EdgetLost) -> Unit Delay20/1
  Unit Delay24/1 -> VisLineFilter4/17(EdgeA2K1)
  VisLineFilter4/1(EdgeSts) -> [LineValid], Unit Delay26/1
  Unit Delay23/1 -> VisLineFilter4/18(EdgeA1K1)
  VisLineFilter4/2(EdgeA3) -> MATLAB Function/1(A3), Unit Delay25/1
  VisLineFilter4/3(EdgeA2) -> MATLAB Function/2(A2), Unit Delay24/1
  [vRef] -> VisLineFilter4/14(vRef)
  Unit Delay20/1 -> VisLineFilter4/21(EdgetLostK1)
  VisLineFilter4/4(EdgeA1) -> MATLAB Function/3(A1), Unit Delay23/1
  [dDeltaX] -> VisLineFilter4/10(dDeltaX)
  [VisEdgeA3] -> VisLineFilter4/3(a3)
  Unit Delay21/1 -> VisLineFilter4/20(EdgeRangeK1)
  VisLineFilter4/5(EdgeA0) -> MATLAB Function/4(A0), Unit Delay22/1
  [dDeltaY] -> VisLineFilter4/11(dDeltaY)
  [VisEdgeA1] -> VisLineFilter4/5(a1)
  [CosOfPsi] -> VisLineFilter4/12(CosOfPsi)
  CalcEgoVehMove/1(dDeltaX) -> [dDeltaX]
  Bus Selector1/1 -> CalcEgoVehMove/2(Kap)  "<Kap>"
  CalcEgoVehMove/3(CosOfPsi) -> [CosOfPsi]
  CalcEgoVehMove/4(SinOfPsi) -> [SinOfPsi]
  Bus Selector1/3 -> CalcEgoVehMove/4(alpSideSlipAngle)  "<alpSideSlipAngle>"
  Bus Selector1/2 -> CalcEgoVehMove/3(Vego), [vRef]  "<VehicleSpd_ms>"
  LaneValid/1 -> Bus Selector/1
  Bus Creator13/1 -> [Left_Lane]  "Left_Lane"
  [Left_Lane] -> Bus Creator7/1
  [Right_Lane] -> Bus Creator7/2
  [Left_RE] -> Bus Creator7/3
  [Right_RE] -> Bus Creator7/4
  Bus Creator7/1 -> HLane/1
  Selector5/1 -> Bus Creator1/1  "Valid"
  Selector7/1 -> Bus Creator3/1  "Valid"
  [LineValid] -> Selector4/1
  Selector4/1 -> Bus Creator13/1  "Valid"
  [LineValid] -> Selector5/1
  Selector6/1 -> Bus Creator2/1  "Valid"
  [LineValid] -> Selector6/1
  [LineValid] -> Selector7/1
  MATLAB Function/1(LeftLane) -> [Leftline]
  MATLAB Function/2(RightLane) -> [Rightline]
  MATLAB Function/3(LeftRe) -> [ReLeftline]
  MATLAB Function/4(RightRe) -> [ReRightline]
